simulink subsystem "Energies_and_Simouts"  (R2021a)
settings: Solver=VariableStepAuto  StartTime=0.0  StopTime=10.0  RelTol=1e-3
values from neighbouring files (symbols this model uses):
  dc_voltage = 600    [battery_parameters.m]
settings Model: Creator=OMISTAJA  LastModifiedBy=OMISTAJA

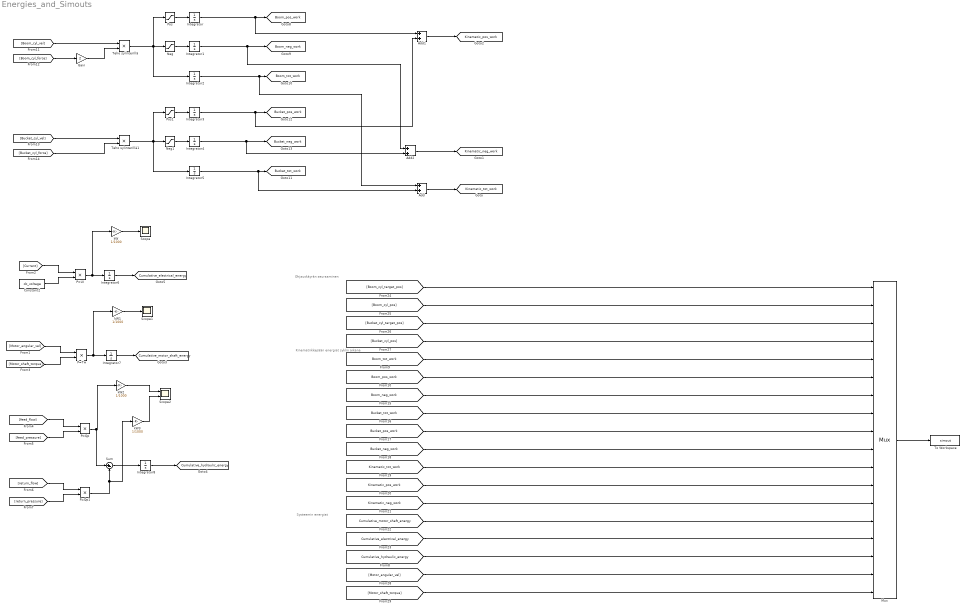
== system Energies_and_Simouts ==
  note: Kinematiikkapään energiat syklin aikana
  note: Ohjauskäyrän seuraaminen
  note: Systeemin energiat
  Add : Sum
  Add1 : Sum
  Add2 : Sum
  Constant2 : Constant  Value=dc_voltage
  Gain : Gain  Gain=2
  Integrator{,1..8} (9 alike) : Integrator
  Mux : Mux  Inputs=18
  Neg : Saturate  UpperLimit=0  LowerLimit=-inf
  Neg1 : Saturate  UpperLimit=0  LowerLimit=-inf
  P=Qp : Product
  P=Qp1 : Product
  P=Tw : Product
  P=UI : Product
  Pos : Saturate  UpperLimit=inf  LowerLimit=0
  Pos1 : Saturate  UpperLimit=inf  LowerLimit=0
  Scope : Scope
  Scope1 : Scope
  Scope2 : Scope  NumInputPorts=2
  Sum : Sum  Inputs=|+-
  Teho sylinterillä : Product
  Teho sylinterillä1 : Product
  To Workspace : ToWorkspace  VariableName=simout  SaveFormat=Structure With Time  SampleTime=-1
  kW{,1..3} (4 alike) : Gain  Gain=1/1000
  tag scope: Boom_neg_work=global, Boom_pos_work=global, Boom_tot_work=global, Bucket_neg_work=global, Bucket_pos_work=global, Bucket_tot_work=global, Cumulative_electrical_energy=global, Cumulative_hydraulic_energy=global, Cumulative_motor_shaft_energy=global, Kinematic_neg_work=global, Kinematic_pos_work=global, Kinematic_tot_work=global
  wires:
  Teho sylinterillä/1 -> Integrator2/1, Neg/1, Pos/1
  [Bucket_cyl_force] -> Teho sylinterillä1/2
  Neg1/1 -> Integrator4/1
  Integrator5/1 -> [Bucket_tot_work], Add/2
  [Boom_cyl_vel] -> Teho sylinterillä/1
  Integrator1/1 -> [Boom_neg_work], Add2/1
  Pos/1 -> Integrator/1
  Neg/1 -> Integrator1/1
  [Bucket_cyl_vel] -> Teho sylinterillä1/1
  Teho sylinterillä1/1 -> Neg1/1, Pos1/1, Integrator5/1
  Pos1/1 -> Integrator3/1
  [Boom_cyl_force] -> Gain/1
  Integrator2/1 -> [Boom_tot_work], Add/1
  Integrator/1 -> [Boom_pos_work], Add1/1
  Integrator4/1 -> [Bucket_neg_work], Add2/2
  Integrator3/1 -> [Bucket_pos_work], Add1/2
  Add/1 -> [Kinematic_tot_work]
  Add2/1 -> [Kinematic_neg_work]
  Add1/1 -> [Kinematic_pos_work]
  Gain/1 -> Teho sylinterillä/2
  [Motor_angular_vel] -> P=Tw/1
  P=Qp1/1 -> Sum/2, kW3/1
  Integrator7/1 -> [Cumulative_motor_shaft_energy]
  [Current] -> P=UI/1
  P=Qp/1 -> kW2/1, Sum/1
  Constant2/1 -> P=UI/2
  [return_pressure] -> P=Qp1/2
  [Motor_shaft_torque] -> P=Tw/2
  Integrator8/1 -> [Cumulative_hydraulic_energy]
  kW3/1 -> Scope2/2
  kW2/1 -> Scope2/1
  [return_flow] -> P=Qp1/1
  Sum/1 -> Integrator8/1
  P=Tw/1 -> Integrator7/1, kW1/1
  P=UI/1 -> Integrator6/1, kW/1
  [feed_pressure] -> P=Qp/2
  [feed_flow] -> P=Qp/1
  kW/1 -> Scope/1
  Integrator6/1 -> [Cumulative_electrical_energy]
  kW1/1 -> Scope1/1
  [Kinematic_pos_work] -> Mux/12
  [Bucket_pos_work] -> Mux/9
  [Cumulative_hydraulic_energy] -> Mux/16
  [Cumulative_motor_shaft_energy] -> Mux/14
  [Kinematic_neg_work] -> Mux/13
  [Bucket_neg_work] -> Mux/10
  [Boom_cyl_target_pos] -> Mux/1
  [Bucket_cyl_target_pos] -> Mux/3
  [Boom_cyl_pos] -> Mux/2
  Mux/1 -> To Workspace/1
  [Boom_neg_work] -> Mux/7
  [Bucket_cyl_pos] -> Mux/4
  [Bucket_tot_work] -> Mux/8
  [Cumulative_electrical_energy] -> Mux/15
  [Boom_tot_work] -> Mux/5
  [Kinematic_tot_work] -> Mux/11
  [Boom_pos_work] -> Mux/6
  [Motor_angular_vel] -> Mux/17
  [Motor_shaft_torque] -> Mux/18
